simulink model "Beobachter_diskret_1D_Model"  (R2016b)
settings: Solver=FixedStepAuto  StartTime=0.0  StopTime=100  FixedStep=0.001  RelTol=1e-3
values from neighbouring files (symbols this model uses):
  A = [0, 1, 0; (m*g*l_C)/I_G, (-C_phi-C_psi)/I_G, C_psi/I_G; 0, C_psi/I_R, -C_psi/I_R]    [Beobachter_1D_diskret.m]    (also in Beobachter_3D_diskret.m = [zeros(3,3), g_LA, zeros(3,3))
  Ad = mySS.A    [Beobachter_1D_diskret.m]    (also in Beobachter_3D_diskret.m = minSYSd.A)
  alpha_M = 0.3    [KF_3D_linear.m]
  B = [0; -1/I_G; 1/I_R]    [Beobachter_1D_diskret.m]    (also in Beobachter_3D_diskret.m = [zeros(3,3); -I_K_inv; I_R_inv])
  Bd = mySS.B    [Beobachter_1D_diskret.m]    (also in Beobachter_3D_diskret.m = minSYSd.B)
  C = [0, 1, 0;0,0,1]    [Beobachter_1D_diskret.m]    (also in Beobachter_3D_diskret.m = [zeros(3,3),eye(3), eye(3)])
  Cd = mySS.C    [Beobachter_1D_diskret.m]    (also in Beobachter_3D_diskret.m = minSYSd.C)
  k = lqrd(A, B, Q, R, Ta)    [Beobachter_1D_diskret.m]
  Ld = (place(Ad', Cd', ew_beo))'    [Beobachter_1D_diskret.m]    (also in Beobachter_3D_diskret.m)
  P_P_0 = eye(3)    [Beobachter_1D_diskret.m]
  R = eye(2)*y_noise(1)/Ta    [Beobachter_1D_diskret.m]    (also in Beobachter_3D_diskret.m = eye(3)*(T_max^(-2)))
  Ta = 0.02    [Beobachter_1D_diskret.m]
  x_0 = degtorad([5;0;0])    [Beobachter_1D_diskret.m]    (also in KF_3D_linear.m = [ [-6.3118;-4.9313;-5.6638]+9.81/sqrt(3);zeros(6,1) ])
  x_0_off = zeros(3,1)    [Beobachter_1D_diskret.m]
undefined symbols (not defined in the file or in its folder): Ld1
libraries: dspindex x3, simulink x1
settings Model: Creator=michael  LastModifiedBy=michael

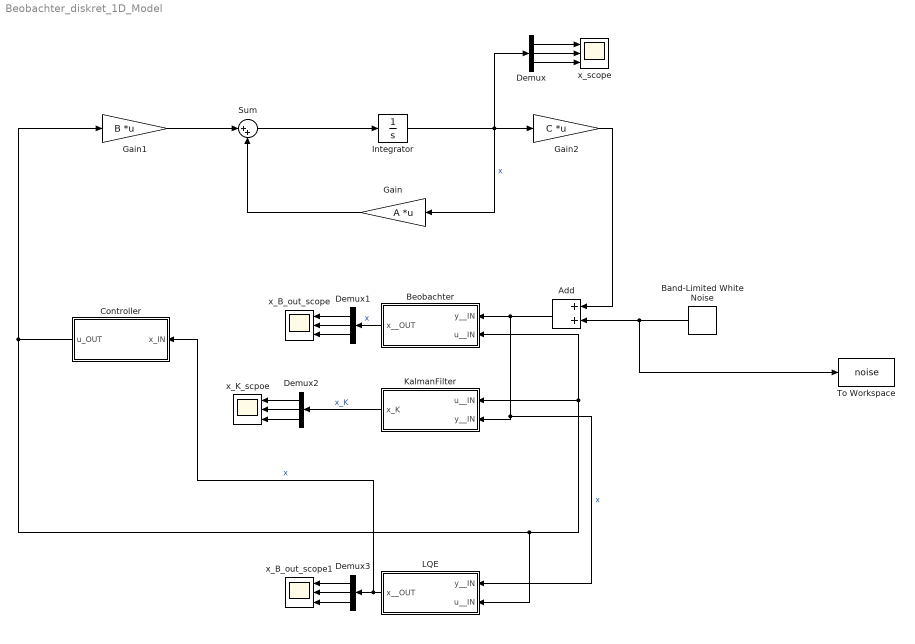
== system Beobachter_diskret_1D_Model ==
  Add : Sum
  Band-Limited White Noise : simulink/Sources/Band-Limited White Noise  Cov=y_noise  Ts=0.02  seed=[23341, 23113]
  Beobachter : Subsystem
  Controller : Subsystem
  Demux{,1..3} (4 alike) : Demux  Outputs=3
  Gain : Gain  Gain=A  Multiplication=Matrix(K*u) (u vector)
  Gain1 : Gain  Gain=B  Multiplication=Matrix(K*u) (u vector)
  Gain2 : Gain  Gain=C  Multiplication=Matrix(K*u) (u vector)
  Integrator : Integrator  InitialCondition=x_0
  KalmanFilter : Subsystem
  LQE : Subsystem
  Sum : Sum  Inputs=|++
  To Workspace : ToWorkspace  VariableName=noise  SaveFormat=Timeseries  SampleTime=-1
  x_B_out_scope : Scope  NumInputPorts=3
  x_B_out_scope1 : Scope  NumInputPorts=3
  x_K_scpoe : Scope  NumInputPorts=3
  x_scope : Scope  NumInputPorts=3
  wires:
  Sum/1 -> Integrator/1
  Gain/1 -> Sum/2
  Gain1/1 -> Sum/1
  Integrator/1 -> Demux/1, Gain/1, Gain2/1  "x"
  Demux/2 -> x_scope/2
  Demux/3 -> x_scope/3
  Demux/1 -> x_scope/1
  Demux1/2 -> x_B_out_scope/2
  Demux1/3 -> x_B_out_scope/3
  Demux1/1 -> x_B_out_scope/1
  Beobachter/1(x__OUT) -> Demux1/1  "x"
  Gain2/1 -> Add/1
  Band-Limited White Noise/1 -> To Workspace/1, Add/2
  Add/1 -> LQE/1(y__IN), KalmanFilter/2(y__IN), Beobachter/1(y__IN)  "x"
  Demux2/2 -> x_K_scpoe/2
  Demux2/3 -> x_K_scpoe/3
  Demux2/1 -> x_K_scpoe/1
  KalmanFilter/1(x_K) -> Demux2/1  "x_K"
  Controller/1(u_OUT) -> LQE/2(u__IN), KalmanFilter/1(u__IN), Beobachter/2(u__IN), Gain1/1
  Demux3/2 -> x_B_out_scope1/2
  Demux3/3 -> x_B_out_scope1/3
  Demux3/1 -> x_B_out_scope1/1
  LQE/1(x__OUT) -> Controller/1(x_IN), Demux3/1  "x"

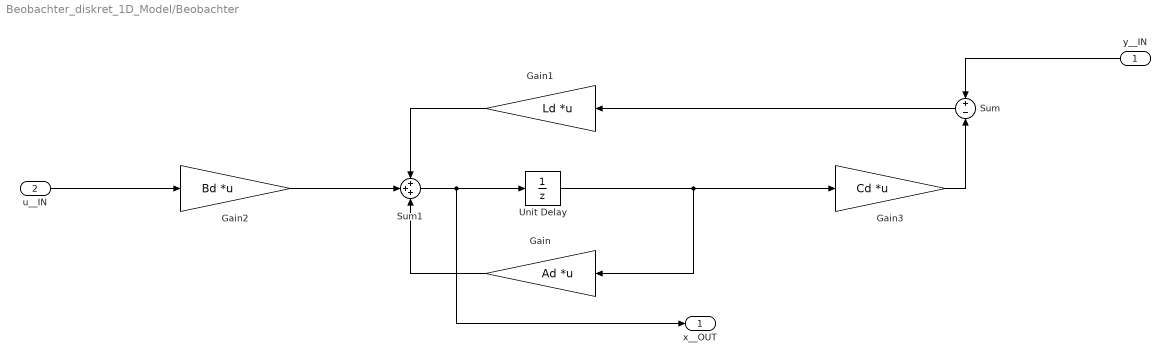
== system Beobachter_diskret_1D_Model/Beobachter ==
  y__IN : Inport  SampleTime=Ta
  u__IN : Inport  Port=2  SampleTime=Ta
  Gain : Gain  Gain=Ad  Multiplication=Matrix(K*u) (u vector)
  Gain1 : Gain  Gain=Ld  Multiplication=Matrix(K*u) (u vector)
  Gain2 : Gain  Gain=Bd  Multiplication=Matrix(K*u) (u vector)
  Gain3 : Gain  Gain=Cd  Multiplication=Matrix(K*u) (u vector)
  Sum : Sum  Inputs=+|-
  Sum1 : Sum  Inputs=+++
  Unit Delay : UnitDelay  InitialCondition=(x_0+x_0_off)  SampleTime=Ta
  x__OUT : Outport
  wires:
  y__IN/1 -> Sum/1
  Sum/1 -> Gain1/1
  Gain2/1 -> Sum1/2
  Gain1/1 -> Sum1/1
  Gain/1 -> Sum1/3
  Gain3/1 -> Sum/2
  Unit Delay/1 -> Gain3/1, Gain/1
  u__IN/1 -> Gain2/1
  Sum1/1 -> x__OUT/1, Unit Delay/1

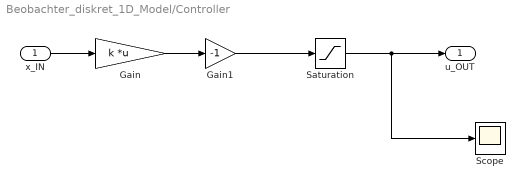
== system Beobachter_diskret_1D_Model/Controller ==
  x_IN : Inport  SampleTime=Ta
  Gain : Gain  Gain=k  Multiplication=Matrix(K*u) (u vector)
  Gain1 : Gain  Gain=-1
  Saturation : Saturate  UpperLimit=0.07  LowerLimit=-0.07
  Scope : Scope
  u_OUT : Outport
  wires:
  x_IN/1 -> Gain/1
  Gain/1 -> Gain1/1
  Gain1/1 -> Saturation/1
  Saturation/1 -> Scope/1, u_OUT/1

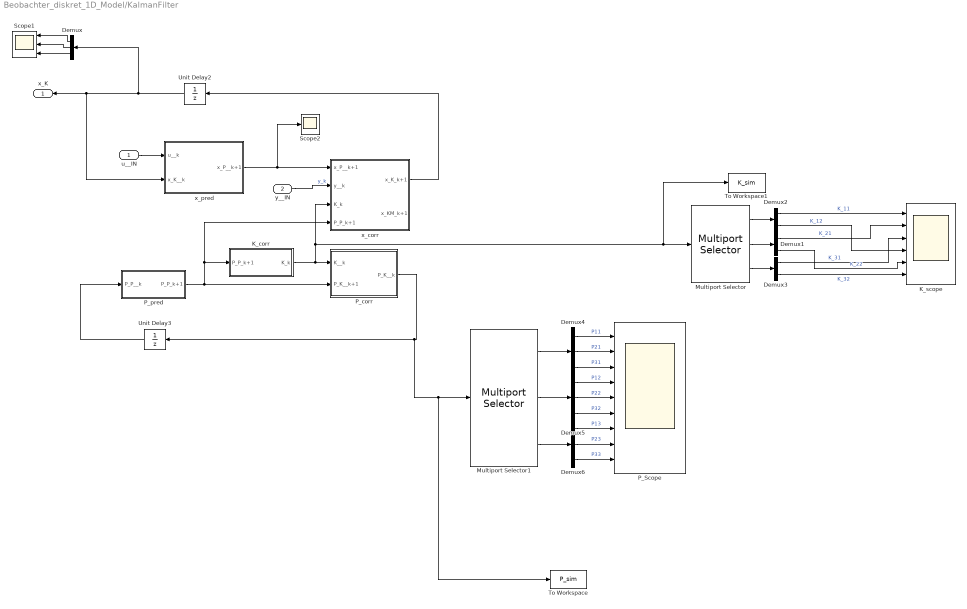
== system Beobachter_diskret_1D_Model/KalmanFilter ==
  u__IN : Inport  SampleTime=0.02
  y__IN : Inport  Port=2  SampleTime=0.02
  Demux{,4..6} (4 alike) : Demux  Outputs=3
  Demux1 : Demux  Outputs=2
  Demux2 : Demux  Outputs=2
  Demux3 : Demux  Outputs=2
  K_corr : Subsystem
  K_scope : Scope  NumInputPorts=6
  Multiport Selector : dspindex/Multiport Selector  rowsOrCols=Rows  idxCellArray={1, 2, 3}  idxErrMode=Clip Index
  Multiport Selector1 : dspindex/Multiport Selector  rowsOrCols=Columns  idxCellArray={1, 2, 3}  idxErrMode=Clip Index
  P_Scope : Scope  NumInputPorts=9
  P_corr : Subsystem
  P_pred : Subsystem
  Scope1 : Scope  NumInputPorts=3
  Scope2 : Scope
  To Workspace : ToWorkspace  VariableName=P_sim  SaveFormat=Timeseries  SampleTime=-1
      settings: MaxDataPoints=1
  To Workspace1 : ToWorkspace  VariableName=K_sim  SaveFormat=Timeseries  SampleTime=-1
      settings: MaxDataPoints=1
  Unit Delay2 : UnitDelay  InitialCondition=x_0  SampleTime=0.02
  Unit Delay3 : UnitDelay  InitialCondition=P_P_0  SampleTime=0.02
  x_corr : Subsystem
  x_pred : Subsystem
  x_K : Outport
  wires:
  x_pred/1(x_P__k+1) -> Scope2/1, x_corr/1(x_P__k+1)
  y__IN/1 -> x_corr/2(y__k)  "y_k"
  P_pred/1(P_P_k+1) -> P_corr/2(P_K__k+1), x_corr/4(P_P_k+1), K_corr/1(P_P_k+1)
  Unit Delay3/1 -> P_pred/1(P_P__k)
  K_corr/1(K_k) -> x_corr/3(K_k), To Workspace1/1, Multiport Selector/1, P_corr/1(K__k)
  u__IN/1 -> x_pred/1(u__k)
  Unit Delay2/1 -> Demux/1, x_K/1, x_pred/2(x_K__k)
  Demux/1 -> Scope1/1
  Demux/2 -> Scope1/2
  Demux/3 -> Scope1/3
  Multiport Selector/2 -> Demux1/1
  Multiport Selector/1 -> Demux2/1
  Multiport Selector/3 -> Demux3/1
  Demux2/1 -> K_scope/1  "K_11"
  Demux2/2 -> K_scope/4  "K_12"
  Demux1/1 -> K_scope/2  "K_21"
  Demux3/2 -> K_scope/6  "K_32"
  Demux3/1 -> K_scope/3  "K_31"
  Demux1/2 -> K_scope/5  "K_22"
  Multiport Selector1/1 -> Demux4/1
  Multiport Selector1/3 -> Demux6/1
  Demux4/1 -> P_Scope/1  "P11"
  Demux4/2 -> P_Scope/2  "P21"
  Demux4/3 -> P_Scope/3  "P31"
  Demux5/1 -> P_Scope/4  "P12"
  Demux5/2 -> P_Scope/5  "P22"
  Demux5/3 -> P_Scope/6  "P32"
  Demux6/1 -> P_Scope/7  "P13"
  Demux6/2 -> P_Scope/8  "P23"
  Demux6/3 -> P_Scope/9  "P33"
  Multiport Selector1/2 -> Demux5/1
  P_corr/1(P_K__k) -> To Workspace/1, Multiport Selector1/1, Unit Delay3/1
  x_corr/1(x_K_k+1) -> Unit Delay2/1

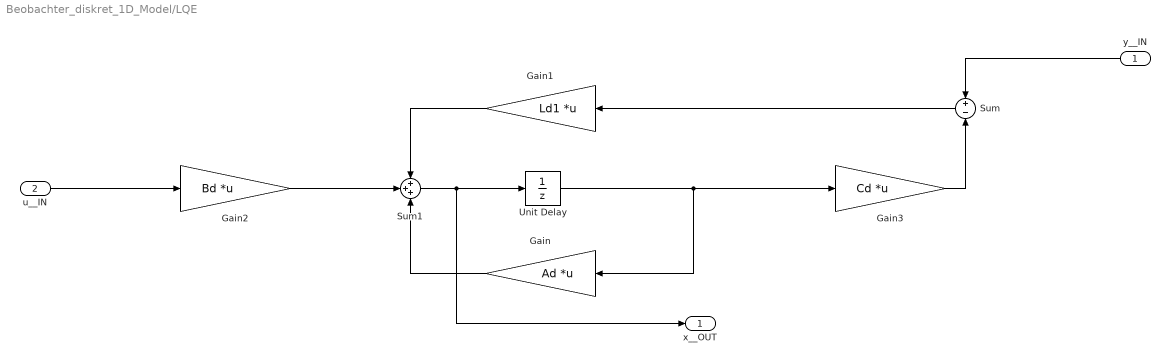
== system Beobachter_diskret_1D_Model/LQE ==
  y__IN : Inport  SampleTime=Ta
  u__IN : Inport  Port=2  SampleTime=Ta
  Gain : Gain  Gain=Ad  Multiplication=Matrix(K*u) (u vector)
  Gain1 : Gain  Gain=Ld1  Multiplication=Matrix(K*u) (u vector)
  Gain2 : Gain  Gain=Bd  Multiplication=Matrix(K*u) (u vector)
  Gain3 : Gain  Gain=Cd  Multiplication=Matrix(K*u) (u vector)
  Sum : Sum  Inputs=+|-
  Sum1 : Sum  Inputs=+++
  Unit Delay : UnitDelay  InitialCondition=(x_0+x_0_off)  SampleTime=Ta
  x__OUT : Outport
  wires:
  Sum1/1 -> Unit Delay/1, x__OUT/1
  u__IN/1 -> Gain2/1
  Unit Delay/1 -> Gain/1, Gain3/1
  Gain3/1 -> Sum/2
  Gain/1 -> Sum1/3
  Gain1/1 -> Sum1/1
  Gain2/1 -> Sum1/2
  Sum/1 -> Gain1/1
  y__IN/1 -> Sum/1

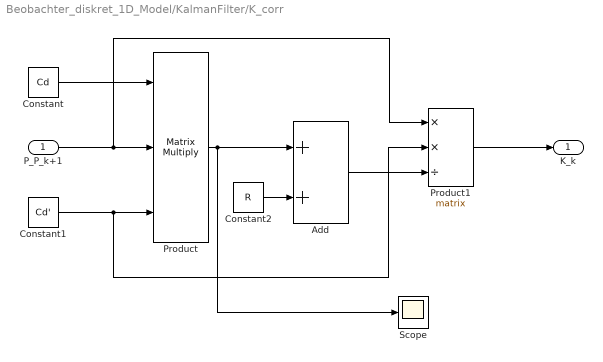
== system Beobachter_diskret_1D_Model/KalmanFilter/K_corr ==
  P_P_k+1 : Inport
  Add : Sum
  Constant : Constant  Value=Cd
  Constant1 : Constant  Value=Cd'
  Constant2 : Constant  Value=R
  Product : Product  Inputs=3  Multiplication=Matrix(*)
  Product1 : Product  Inputs=**/  Multiplication=Matrix(*)
  Scope : Scope
  K_k : Outport
  wires:
  Constant/1 -> Product/1
  P_P_k+1/1 -> Product1/1, Product/2
  Constant1/1 -> Product1/2, Product/3
  Constant2/1 -> Add/2
  Product/1 -> Scope/1, Add/1
  Add/1 -> Product1/3
  Product1/1 -> K_k/1

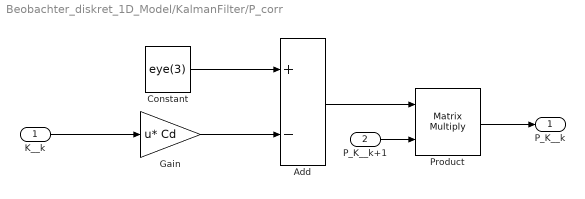
== system Beobachter_diskret_1D_Model/KalmanFilter/P_corr ==
  K__k : Inport
  P_K__k+1 : Inport  Port=2
  Add : Sum  Inputs=+-
  Constant : Constant  Value=eye(3)
  Gain : Gain  Gain=Cd  Multiplication=Matrix(u*K)
  Product : Product  Multiplication=Matrix(*)
  P_K__k : Outport
  wires:
  K__k/1 -> Gain/1
  Constant/1 -> Add/1
  Gain/1 -> Add/2
  Add/1 -> Product/1
  P_K__k+1/1 -> Product/2
  Product/1 -> P_K__k/1

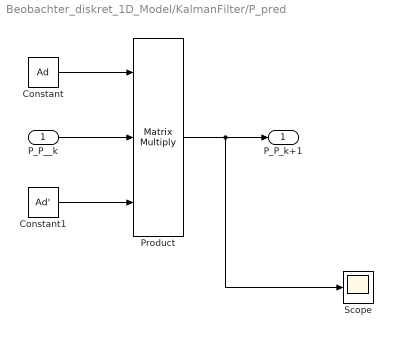
== system Beobachter_diskret_1D_Model/KalmanFilter/P_pred ==
  P_P__k : Inport
  Constant : Constant  Value=Ad
  Constant1 : Constant  Value=Ad'
  Product : Product  Inputs=3  Multiplication=Matrix(*)
  Scope : Scope
  P_P_k+1 : Outport
  wires:
  Constant1/1 -> Product/3
  P_P__k/1 -> Product/2
  Constant/1 -> Product/1
  Product/1 -> Scope/1, P_P_k+1/1

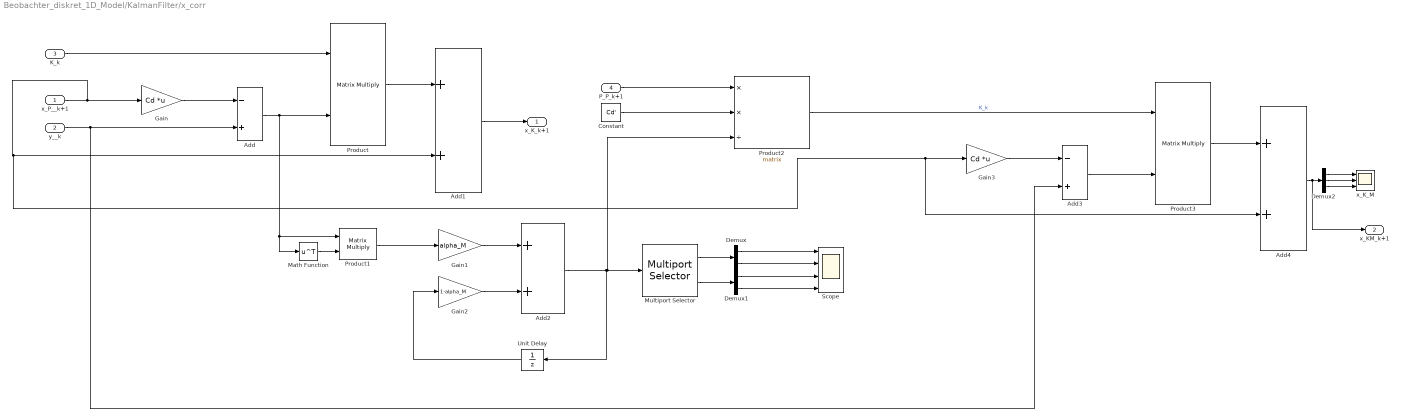
== system Beobachter_diskret_1D_Model/KalmanFilter/x_corr ==
  x_P__k+1 : Inport
  y__k : Inport  Port=2
  K_k : Inport  Port=3
  P_P_k+1 : Inport  Port=4
  Add : Sum  Inputs=-+
  Add1 : Sum
  Add2 : Sum
  Add3 : Sum  Inputs=-+
  Add4 : Sum
  Constant : Constant  Value=Cd'
  Demux : Demux  Outputs=2
  Demux1 : Demux  Outputs=2
  Demux2 : Demux  Outputs=3
  Gain : Gain  Gain=Cd  Multiplication=Matrix(K*u) (u vector)
  Gain1 : Gain  Gain=alpha_M
  Gain2 : Gain  Gain=1-alpha_M
  Gain3 : Gain  Gain=Cd  Multiplication=Matrix(K*u) (u vector)
  Math Function : Math  Operator=transpose  SaturateOnIntegerOverflow=on
  Multiport Selector : dspindex/Multiport Selector  rowsOrCols=Columns  idxCellArray={1,2}  idxErrMode=Clip Index
  Product : Product  Multiplication=Matrix(*)
  Product1 : Product  Multiplication=Matrix(*)
  Product2 : Product  Inputs=**/  Multiplication=Matrix(*)
  Product3 : Product  Multiplication=Matrix(*)
  Scope : Scope  NumInputPorts=4
  Unit Delay : UnitDelay  InitialCondition=zeros(2,2)  SampleTime=-1
  x_K_M : Scope  NumInputPorts=3
  x_K_k+1 : Outport
  x_KM_k+1 : Outport  Port=2
  wires:
  Gain/1 -> Add/1
  K_k/1 -> Product/1
  Add/1 -> Product/2, Math Function/1, Product1/1
  Product/1 -> Add1/1
  Add1/1 -> x_K_k+1/1
  Math Function/1 -> Product1/2
  Product1/1 -> Gain1/1
  Gain1/1 -> Add2/1
  Gain2/1 -> Add2/2
  Add2/1 -> Product2/3, Multiport Selector/1, Unit Delay/1
  Unit Delay/1 -> Gain2/1
  Multiport Selector/2 -> Demux1/1
  Demux/1 -> Scope/1
  Demux/2 -> Scope/2
  Demux1/1 -> Scope/3
  Demux1/2 -> Scope/4
  Multiport Selector/1 -> Demux/1
  Constant/1 -> Product2/2
  x_P__k+1/1 -> Add4/2, Gain3/1, Add1/2, Gain/1
  Gain3/1 -> Add3/1
  y__k/1 -> Add3/2, Add/2
  Add3/1 -> Product3/2
  Product3/1 -> Add4/1
  Product2/1 -> Product3/1  "K_k"
  Add4/1 -> x_KM_k+1/1, Demux2/1
  Demux2/1 -> x_K_M/1
  Demux2/2 -> x_K_M/2
  Demux2/3 -> x_K_M/3
  P_P_k+1/1 -> Product2/1

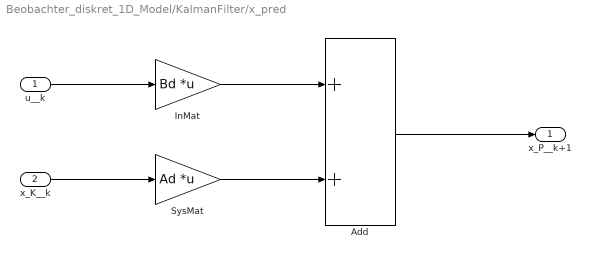
== system Beobachter_diskret_1D_Model/KalmanFilter/x_pred ==
  u__k : Inport
  x_K__k : Inport  Port=2
  Add : Sum
  InMat : Gain  Gain=Bd  Multiplication=Matrix(K*u) (u vector)
  SysMat : Gain  Gain=Ad  Multiplication=Matrix(K*u) (u vector)
  x_P__k+1 : Outport
  wires:
  u__k/1 -> InMat/1
  x_K__k/1 -> SysMat/1
  SysMat/1 -> Add/2
  InMat/1 -> Add/1
  Add/1 -> x_P__k+1/1
